simulink model "EfficiencySensitivityAnalysis"  (R2024b)
settings: Solver=FixedStepAuto  StartTime=0.0  StopTime=451.4  FixedStep=0.1  RelTol=1e-3
values from neighbouring files (symbols this model uses):
  GR = 6    [EfficiencySensitivityAnalysisParameters.m]
  mu_gb = 0.95    [EfficiencySensitivityAnalysisParameters.m]
  phi = 0    [EfficiencySensitivityAnalysisParameters.m]
  Tinit = 40    [EfficiencySensitivityAnalysisParameters.m]
  Tr = 0.33    [EfficiencySensitivityAnalysisParameters.m]
(part 3 of 3)

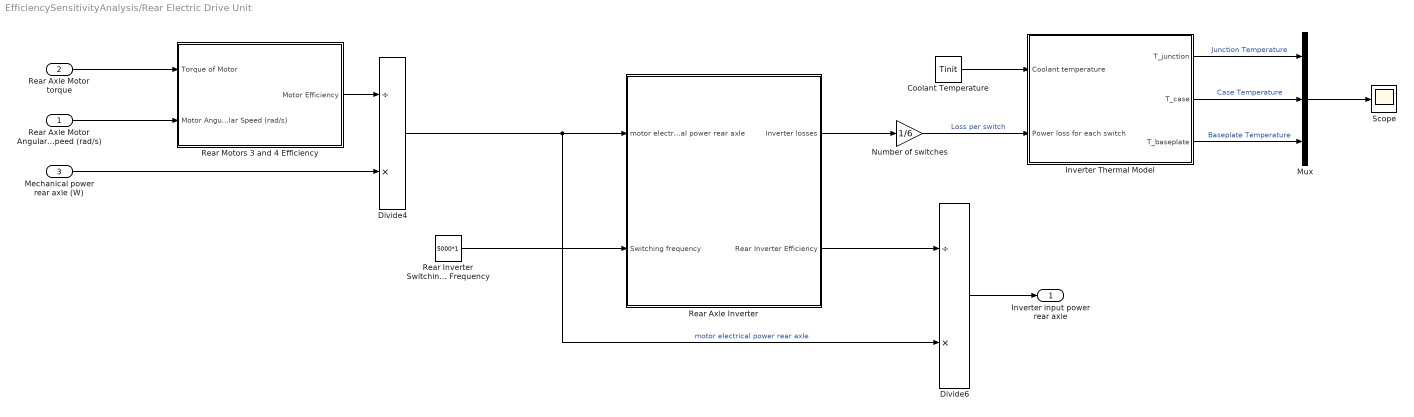
== system EfficiencySensitivityAnalysis/Rear Electric Drive Unit ==
  Rear Axle Motor Angular Speed (rad/s) : Inport
  Rear Axle Motor torque : Inport  Port=2
  Mechanical power rear axle (W) : Inport  Port=3
  Coolant Temperature : Constant  Value=Tinit
  Divide4 : Product  Inputs=/*
  Divide6 : Product  Inputs=/*
  Inverter Thermal Model : Subsystem
  Mux : Mux  Inputs=3
  Number of switches : Gain  Gain=1/6
  Rear Axle Inverter : Subsystem
  Rear Inverter Switching Frequency : Constant  Value=5000*1
  Rear Motors 3 and 4 Efficiency : Subsystem
  Scope : Scope
  Inverter input power rear axle : Outport
  wires:
  Rear Inverter Switching Frequency/1 -> Rear Axle Inverter/2(Switching frequency)
  Rear Axle Motor Angular Speed (rad/s)/1 -> Rear Motors 3 and 4 Efficiency/2(Motor Angular Speed (rad/s))
  Mechanical power rear axle (W)/1 -> Divide4/2
  Divide6/1 -> Inverter input power rear axle/1
  Rear Motors 3 and 4 Efficiency/1(Motor Efficiency) -> Divide4/1
  Rear Axle Motor torque/1 -> Rear Motors 3 and 4 Efficiency/1(Torque of Motor)
  Rear Axle Inverter/2(Rear Inverter Efficiency) -> Divide6/1
  Coolant Temperature/1 -> Inverter Thermal Model/1(Coolant temperature)
  Rear Axle Inverter/1(Inverter losses) -> Number of switches/1
  Number of switches/1 -> Inverter Thermal Model/2(Power loss for each switch)  "Loss per switch"
  Inverter Thermal Model/1(T_junction) -> Mux/1  "Junction Temperature"
  Inverter Thermal Model/2(T_case) -> Mux/2  "Case Temperature"
  Inverter Thermal Model/3(T_baseplate) -> Mux/3  "Baseplate Temperature"
  Mux/1 -> Scope/1
  Divide4/1 -> Divide6/2, Rear Axle Inverter/1(motor electrical power rear axle)  "motor electrical power rear axle"

== system EfficiencySensitivityAnalysis/Battery/Battery Thermal Model ==
  In1 : Inport
  In2 : Inport  Port=2
  1/R_thjc : Gain  Gain=1/0.15
  C_th_junction : Gain  Gain=1/(25*10^4)
  Integrator : Integrator  InitialCondition=25
  Subtract : Sum  Inputs=+-
  Subtract1 : Sum  Inputs=-+
  Battery  temperature : Outport
  wires:
  In2/1 -> Subtract1/2
  C_th_junction/1 -> Integrator/1
  Subtract1/1 -> C_th_junction/1
  Integrator/1 -> Battery  temperature/1, Subtract/1  "Battery  temperature"
  In1/1 -> Subtract/2
  Subtract/1 -> 1/R_thjc/1
  1/R_thjc/1 -> Subtract1/1

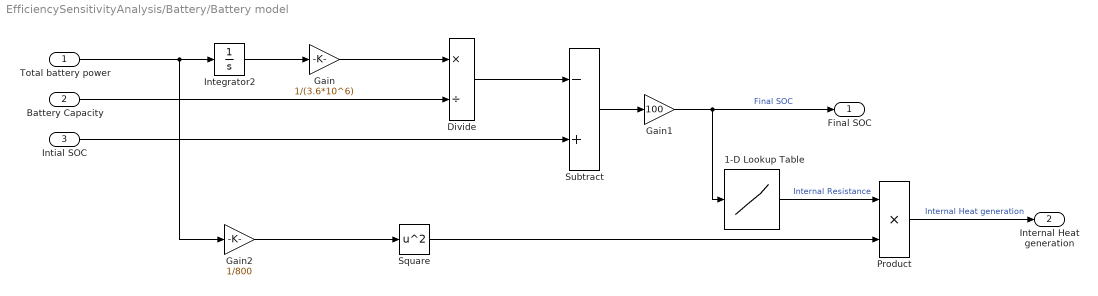
== system EfficiencySensitivityAnalysis/Battery/Battery model ==
  Total battery power : Inport
  Battery Capacity : Inport  Port=2
  Intial SOC : Inport  Port=3
  1-D Lookup Table : Lookup_n-D  NumberOfTableDimensions=1  BreakpointsForDimension1=[1 10 20 30 40 50 60 70 80 90 99]  Table=[0.038 0.037 0.0365 0.036 0.0357 0.035 0.0347 0.0343 0.0342 0.0342 0.035]  InternalRulePriority=Speed  RndMeth=Simplest
  Divide : Product  Inputs=*/
  Gain : Gain  Gain=1/(3.6*10^6)
  Gain1 : Gain  Gain=100
  Gain2 : Gain  Gain=1/800
  Integrator2 : Integrator
  Product : Product
  Square : Math  Operator=square
  Subtract : Sum  Inputs=-+
  Final SOC : Outport
  Internal Heat generation : Outport  Port=2
  wires:
  Total battery power/1 -> Gain2/1, Integrator2/1
  Gain1/1 -> 1-D Lookup Table/1, Final SOC/1  "Final SOC"
  Gain/1 -> Divide/1
  Subtract/1 -> Gain1/1
  Battery Capacity/1 -> Divide/2
  Integrator2/1 -> Gain/1
  1-D Lookup Table/1 -> Product/1  "Internal Resistance"
  Square/1 -> Product/2
  Product/1 -> Internal Heat generation/1  "Internal Heat generation"
  Gain2/1 -> Square/1
  Divide/1 -> Subtract/1
  Intial SOC/1 -> Subtract/2

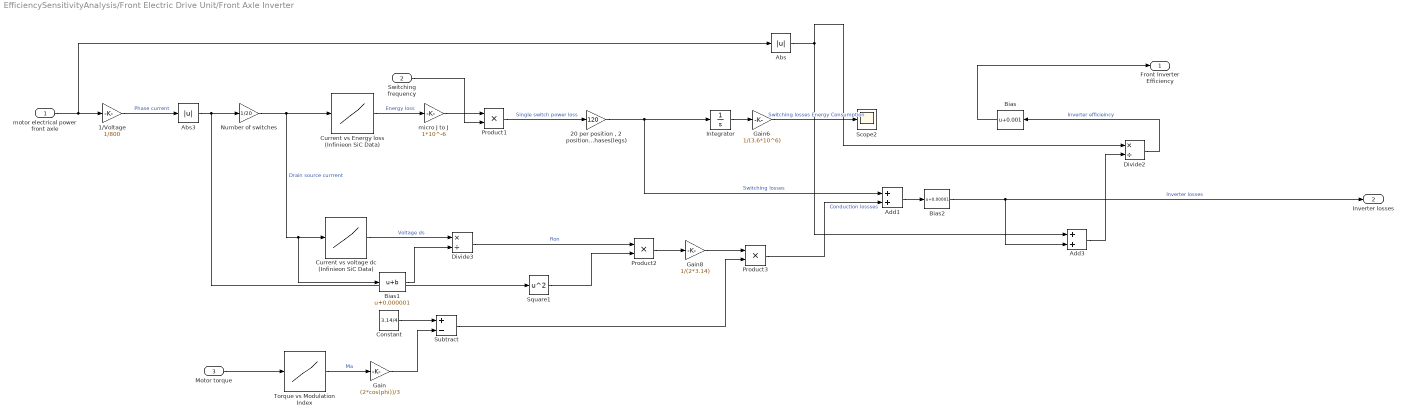
== system EfficiencySensitivityAnalysis/Front Electric Drive Unit/Front Axle Inverter ==
  motor electrical power front axle : Inport
  Switching frequency : Inport  Port=2
  Motor torque : Inport  Port=3
  1/Voltage : Gain  Gain=1/800
  "20 per position , 2 positions and 3 phases(legs)" : Gain  Gain=120
  Abs : Abs  SaturateOnIntegerOverflow=off
  Abs3 : Abs  SaturateOnIntegerOverflow=off
  Add1 : Sum
  Add3 : Sum
  Bias : Bias  Bias=0.001  SaturateOnIntegerOverflow=off
  Bias1 : Bias  Bias=0.000001  SaturateOnIntegerOverflow=off
  Bias2 : Bias  Bias=0.00001  SaturateOnIntegerOverflow=off
  Constant : Constant  Value=3.14/4
  Current vs Energy loss (Infinieon SiC Data) : Lookup_n-D  NumberOfTableDimensions=1  BreakpointsForDimension1=[0;5;10;15;20;25;30;35;40;45;50]  Table=[0;250;300;380;500;600;750;900;1050;1200;1400]  InternalRulePriority=Speed  RndMeth=Simplest
  Current vs voltage dc (Infinieon SiC Data) : Lookup_n-D  NumberOfTableDimensions=1  BreakpointsForDimension1=[20;40;60;80;110]  Table=[1;2;5;8;20]  InternalRulePriority=Speed  RndMeth=Simplest
  Divide2 : Product  Inputs=*/
  Divide3 : Product  Inputs=*/
  Gain : Gain  Gain=(2*cos(phi))/3
  Gain6 : Gain  Gain=1/(3.6*10^6)
  Gain8 : Gain  Gain=1/(2*3.14)
  Integrator : Integrator
  Number of switches : Gain  Gain=1/20
  Product1 : Product
  Product2 : Product
  Product3 : Product
  Scope2 : Scope
  Square1 : Math  Operator=square
  Subtract : Sum  Inputs=+-
  Torque vs Modulation Index : Lookup_n-D  NumberOfTableDimensions=1  BreakpointsForDimension1=[0;100;200;300;400]  Table=[0.3;0.5;0.7;0.8;0.95]  InternalRulePriority=Speed  RndMeth=Simplest
  micro J to J : Gain  Gain=1*10^-6
  Front Inverter Efficiency : Outport
  Inverter losses : Outport  Port=2
  wires:
  Bias/1 -> Front Inverter Efficiency/1
  Switching frequency/1 -> Product1/2
  Integrator/1 -> Gain6/1
  Current vs Energy loss (Infinieon SiC Data)/1 -> micro J to J/1  "Energy loss"
  motor electrical power front axle/1 -> Abs/1, 1/Voltage/1
  Abs/1 -> Divide2/1, Add3/1
  Gain/1 -> Subtract/2
  Add1/1 -> Bias2/1
  Constant/1 -> Subtract/1
  Square1/1 -> Product2/2
  Torque vs Modulation Index/1 -> Gain/1  "Ma"
  Motor torque/1 -> Torque vs Modulation Index/1
  Divide3/1 -> Product2/1  "Ron"
  Divide2/1 -> Bias/1  "Inverter efficieincy"
  Current vs voltage dc (Infinieon SiC Data)/1 -> Divide3/1  "Voltage ds"
  Subtract/1 -> Product3/2
  Number of switches/1 -> Bias1/1, Current vs voltage dc (Infinieon SiC Data)/1, Current vs Energy loss (Infinieon SiC Data)/1  "Drain source currrent"
  Product3/1 -> Add1/2  "Conduction lossses"
  Product2/1 -> Gain8/1
  Add3/1 -> Divide2/2
  Product1/1 -> "20 per position , 2 positions and 3 phases(legs)"/1  "Single switch power loss"
  "20 per position , 2 positions and 3 phases(legs)"/1 -> Integrator/1, Add1/1  "Switching losses"
  micro J to J/1 -> Product1/1
  1/Voltage/1 -> Abs3/1  "Phase current"
  Gain8/1 -> Product3/1
  Bias1/1 -> Divide3/2
  Gain6/1 -> Scope2/1  "Switching losses Energy Consumption"
  Bias2/1 -> Inverter losses/1, Add3/2  "Inverter losses"
  Abs3/1 -> Square1/1, Number of switches/1

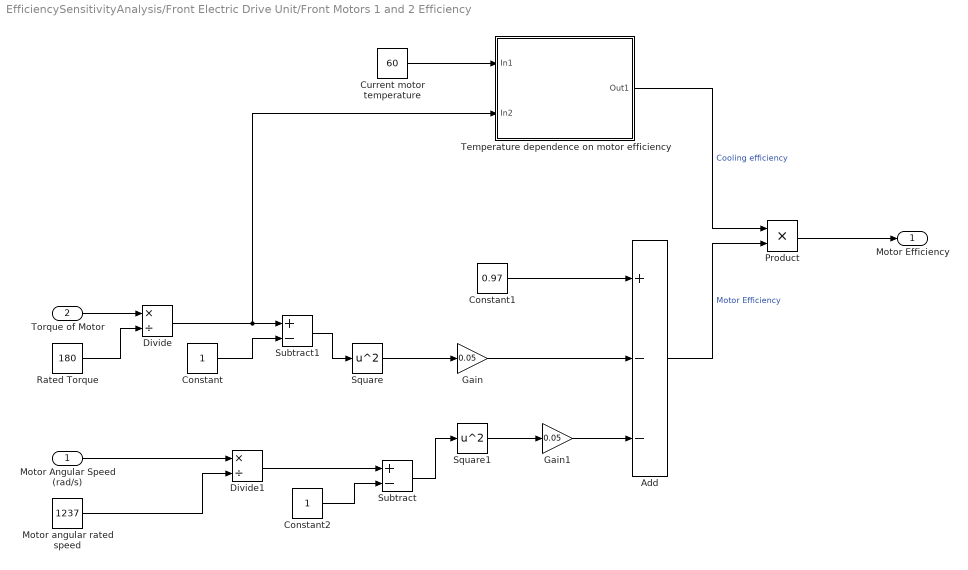
== system EfficiencySensitivityAnalysis/Front Electric Drive Unit/Front Motors 1 and 2 Efficiency  ==
  Motor Angular Speed (rad/s) : Inport
  Torque of Motor : Inport  Port=2
  Add : Sum  Inputs=+--
  Constant : Constant
  Constant1 : Constant  Value=0.97
  Constant2 : Constant
  Current motor temperature : Constant  Value=60
  Divide : Product  Inputs=*/
  Divide1 : Product  Inputs=*/
  Gain : Gain  Gain=0.05
  Gain1 : Gain  Gain=0.05
  Motor angular rated speed : Constant  Value=1237
  Product : Product
  Rated Torque : Constant  Value=180
  Square : Math  Operator=square
  Square1 : Math  Operator=square
  Subtract : Sum  Inputs=+-
  Subtract1 : Sum  Inputs=+-
  Temperature dependence on motor efficiency : Subsystem
  Motor Efficiency : Outport
  wires:
  Constant1/1 -> Add/1
  Square1/1 -> Gain1/1
  Gain/1 -> Add/2
  Constant2/1 -> Subtract/2
  Gain1/1 -> Add/3
  Subtract/1 -> Square1/1
  Motor angular rated speed/1 -> Divide1/2
  Torque of Motor/1 -> Divide/1
  Divide/1 -> Temperature dependence on motor efficiency/2(In2), Subtract1/1
  Square/1 -> Gain/1
  Rated Torque/1 -> Divide/2
  Subtract1/1 -> Square/1
  Current motor temperature/1 -> Temperature dependence on motor efficiency/1(In1)
  Divide1/1 -> Subtract/1
  Constant/1 -> Subtract1/2
  Add/1 -> Product/2  "Motor Efficiency"
  Temperature dependence on motor efficiency/1(Out1) -> Product/1  "Cooling efficiency"
  Motor Angular Speed (rad/s)/1 -> Divide1/1
  Product/1 -> Motor Efficiency/1

== system EfficiencySensitivityAnalysis/Front Electric Drive Unit/Inverter Thermal Model ==
  Coolant temperature : Inport
  Power loss for each switch : Inport  Port=2
  Base plate thermal model : Subsystem
  Case thermal model : Subsystem
  Junction thermal model : Subsystem
  T_junction : Outport
  T_case : Outport  Port=2
  T_baseplate : Outport  Port=3
  wires:
  Junction thermal model/1(Junction temperature) -> Case thermal model/1(Junction temperature), T_junction/1
  Case thermal model/1(Case temperature) -> T_case/1, Base plate thermal model/1(Case temperature), Junction thermal model/1(Case temperature)
  Base plate thermal model/1(Baseplate temperature) -> T_baseplate/1, Case thermal model/2(Base plate temperature)
  Coolant temperature/1 -> Base plate thermal model/2(Coolant temperature)
  Power loss for each switch/1 -> Junction thermal model/2(Power loss for each switch)

== system EfficiencySensitivityAnalysis/Rear Electric Drive Unit/Inverter Thermal Model ==
  Coolant temperature : Inport
  Power loss for each switch : Inport  Port=2
  Base plate thermal model : Subsystem
  Case thermal model : Subsystem
  Junction thermal model : Subsystem
  T_junction : Outport
  T_case : Outport  Port=2
  T_baseplate : Outport  Port=3
  wires:
  Junction thermal model/1(Junction temperature) -> Case thermal model/1(Junction temperature), T_junction/1
  Case thermal model/1(Case temperature) -> T_case/1, Base plate thermal model/1(Case temperature), Junction thermal model/1(Case temperature)
  Base plate thermal model/1(Baseplate temperature) -> T_baseplate/1, Case thermal model/2(Base plate temperature)
  Coolant temperature/1 -> Base plate thermal model/2(Coolant temperature)
  Power loss for each switch/1 -> Junction thermal model/2(Power loss for each switch)

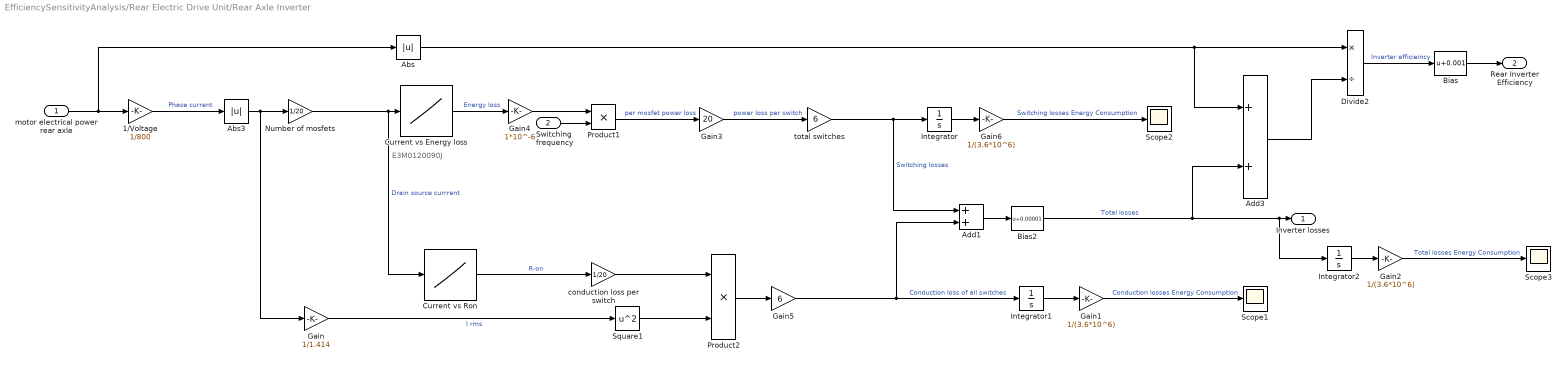
== system EfficiencySensitivityAnalysis/Rear Electric Drive Unit/Rear Axle Inverter ==
  note: E3M0120090J
  motor electrical power rear axle : Inport
  Switching frequency : Inport  Port=2
  1/Voltage : Gain  Gain=1/800
  Abs : Abs  SaturateOnIntegerOverflow=off
  Abs3 : Abs  SaturateOnIntegerOverflow=off
  Add1 : Sum
  Add3 : Sum
  Bias : Bias  Bias=0.001  SaturateOnIntegerOverflow=off
  Bias2 : Bias  Bias=0.00001  SaturateOnIntegerOverflow=off
  "Current vs Energy loss " : Lookup_n-D  NumberOfTableDimensions=1  BreakpointsForDimension1=[5;10;15;20;25;30]  Table=[21;26;32;40;55;70]  InternalRulePriority=Speed  RndMeth=Simplest
  "Current vs Ron " : Lookup_n-D  NumberOfTableDimensions=1  BreakpointsForDimension1=[5;10;15;20;25;30]  Table=[0.15;0.152;0.158;0.165;0.17;0.175]  InternalRulePriority=Speed  RndMeth=Simplest
  Divide2 : Product  Inputs=*/
  Gain : Gain  Gain=1/1.414
  Gain1 : Gain  Gain=1/(3.6*10^6)
  Gain2 : Gain  Gain=1/(3.6*10^6)
  Gain3 : Gain  Gain=20
  Gain4 : Gain  Gain=1*10^-6
  Gain5 : Gain  Gain=6
  Gain6 : Gain  Gain=1/(3.6*10^6)
  Integrator : Integrator
  Integrator1 : Integrator
  Integrator2 : Integrator
  Number of mosfets : Gain  Gain=1/20
  Product1 : Product
  Product2 : Product
  Scope1 : Scope
  Scope2 : Scope
  Scope3 : Scope
  Square1 : Math  Operator=square
  conduction loss per switch : Gain  Gain=1/20
  total switches : Gain  Gain=6
  Inverter losses : Outport
  Rear Inverter Efficiency : Outport  Port=2
  wires:
  Bias/1 -> Rear Inverter Efficiency/1
  Switching frequency/1 -> Product1/2
  Integrator/1 -> Gain6/1
  motor electrical power rear axle/1 -> Abs/1, 1/Voltage/1
  Abs/1 -> Divide2/1, Add3/1
  Add1/1 -> Bias2/1
  Square1/1 -> Product2/2
  Divide2/1 -> Bias/1  "Inverter efficieincy"
  Add3/1 -> Divide2/2
  Product1/1 -> Gain3/1  "per mosfet power loss"
  total switches/1 -> Integrator/1, Add1/1  "Switching losses"
  1/Voltage/1 -> Abs3/1  "Phase current"
  Gain6/1 -> Scope2/1  "Switching losses Energy Consumption"
  Abs3/1 -> Number of mosfets/1, Gain/1
  Integrator1/1 -> Gain1/1
  Gain1/1 -> Scope1/1  "Conduction losses Energy Consumption"
  Product2/1 -> Gain5/1
  Gain2/1 -> Scope3/1  "Total losses Energy Consumption"
  Integrator2/1 -> Gain2/1
  Bias2/1 -> Inverter losses/1, Integrator2/1, Add3/2  "Total losses"
  Gain/1 -> Square1/1  "I rms"
  Gain4/1 -> Product1/1
  Number of mosfets/1 -> "Current vs Ron "/1, "Current vs Energy loss "/1  "Drain source currrent"
  "Current vs Energy loss "/1 -> Gain4/1  "Energy loss"
  "Current vs Ron "/1 -> conduction loss per switch/1  "R-on"
  conduction loss per switch/1 -> Product2/1
  Gain5/1 -> Integrator1/1, Add1/2  "Conduction loss of all switches"
  Gain3/1 -> total switches/1  "power loss per switch"

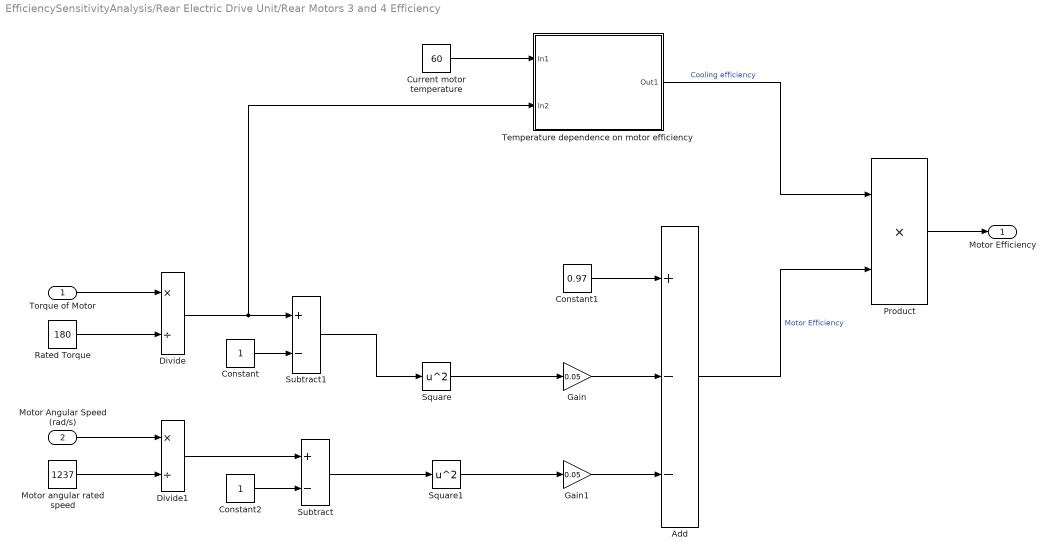
== system EfficiencySensitivityAnalysis/Rear Electric Drive Unit/Rear Motors 3 and 4 Efficiency ==
  Torque of Motor : Inport
  Motor Angular Speed (rad/s) : Inport  Port=2
  Add : Sum  Inputs=+--
  Constant : Constant
  Constant1 : Constant  Value=0.97
  Constant2 : Constant
  Current motor temperature : Constant  Value=60
  Divide : Product  Inputs=*/
  Divide1 : Product  Inputs=*/
  Gain : Gain  Gain=0.05
  Gain1 : Gain  Gain=0.05
  Motor angular rated speed : Constant  Value=1237
  Product : Product
  Rated Torque : Constant  Value=180
  Square : Math  Operator=square
  Square1 : Math  Operator=square
  Subtract : Sum  Inputs=+-
  Subtract1 : Sum  Inputs=+-
  Temperature dependence on motor efficiency : Subsystem
  Motor Efficiency : Outport
  wires:
  Torque of Motor/1 -> Divide/1
  Motor Angular Speed (rad/s)/1 -> Divide1/1
  Subtract/1 -> Square1/1
  Gain/1 -> Add/2
  Constant2/1 -> Subtract/2
  Divide1/1 -> Subtract/1
  Rated Torque/1 -> Divide/2
  Constant/1 -> Subtract1/2
  Constant1/1 -> Add/1
  Gain1/1 -> Add/3
  Motor angular rated speed/1 -> Divide1/2
  Square1/1 -> Gain1/1
  Square/1 -> Gain/1
  Subtract1/1 -> Square/1
  Divide/1 -> Temperature dependence on motor efficiency/2(In2), Subtract1/1
  Temperature dependence on motor efficiency/1(Out1) -> Product/1  "Cooling efficiency"
  Current motor temperature/1 -> Temperature dependence on motor efficiency/1(In1)
  Add/1 -> Product/2  "Motor Efficiency"
  Product/1 -> Motor Efficiency/1

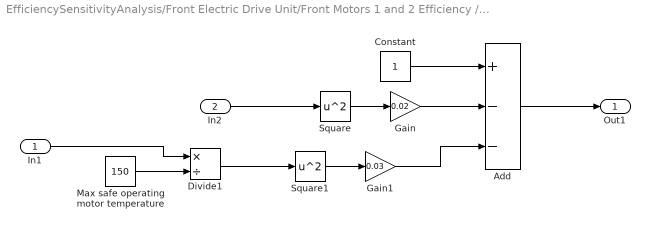
== system EfficiencySensitivityAnalysis/Front Electric Drive Unit/Front Motors 1 and 2 Efficiency /Temperature dependence on motor efficiency ==
  In1 : Inport
  In2 : Inport  Port=2
  Add : Sum  Inputs=+--
  Constant : Constant
  Divide1 : Product  Inputs=*/
  Gain : Gain  Gain=0.02
  Gain1 : Gain  Gain=0.03
  Max safe operating motor temperature : Constant  Value=150
  Square : Math  Operator=square
  Square1 : Math  Operator=square
  Out1 : Outport
  wires:
  Square/1 -> Gain/1
  Square1/1 -> Gain1/1
  In1/1 -> Divide1/1
  Divide1/1 -> Square1/1
  Add/1 -> Out1/1
  Gain1/1 -> Add/3
  Max safe operating motor temperature/1 -> Divide1/2
  Gain/1 -> Add/2
  Constant/1 -> Add/1
  In2/1 -> Square/1

== system EfficiencySensitivityAnalysis/Front Electric Drive Unit/Inverter Thermal Model/Base plate thermal model ==
  Case temperature : Inport
  Coolant temperature : Inport  Port=2
  1/R_thbs : Gain  Gain=1/0.03
  1/R_thcb : Gain  Gain=1/0.015
  Add : Sum  Inputs=+-
  Gain : Gain  Gain=1/100
  Integrator : Integrator  InitialCondition=Tinit
  Subtract : Sum  Inputs=+-
  Subtract1 : Sum  Inputs=+-
  Baseplate temperature : Outport
  wires:
  Integrator/1 -> Subtract/2, Baseplate temperature/1, Subtract1/1  "Baseplate temperature"
  1/R_thcb/1 -> Add/1
  Gain/1 -> Integrator/1
  Subtract/1 -> 1/R_thcb/1
  Case temperature/1 -> Subtract/1
  Coolant temperature/1 -> Subtract1/2
  Subtract1/1 -> 1/R_thbs/1
  1/R_thbs/1 -> Add/2
  Add/1 -> Gain/1

== system EfficiencySensitivityAnalysis/Front Electric Drive Unit/Inverter Thermal Model/Case thermal model ==
  Junction temperature : Inport
  Base plate temperature : Inport  Port=2
  1/R_thcb : Gain  Gain=1/0.015
  1/R_thjc : Gain  Gain=1/0.51
  Gain : Gain  Gain=1/20
  Integrator : Integrator  InitialCondition=Tinit
  Subtract : Sum  Inputs=+-
  Subtract1 : Sum  Inputs=+-
  Subtract2 : Sum  Inputs=+-
  Case temperature : Outport
  wires:
  Subtract1/1 -> Gain/1
  Integrator/1 -> Case temperature/1, Subtract2/1, Subtract/2  "Case temperature"
  Gain/1 -> Integrator/1
  Subtract/1 -> 1/R_thjc/1
  Base plate temperature/1 -> Subtract2/2
  Subtract2/1 -> 1/R_thcb/1
  1/R_thcb/1 -> Subtract1/2
  Junction temperature/1 -> Subtract/1
  1/R_thjc/1 -> Subtract1/1

== system EfficiencySensitivityAnalysis/Front Electric Drive Unit/Inverter Thermal Model/Junction thermal model ==
  Case temperature : Inport
  Power loss for each switch : Inport  Port=2
  1/R_thjc : Gain  Gain=1/0.25
  C_th_junction : Gain  Gain=1/6
  Integrator : Integrator  InitialCondition=Tinit
  Subtract : Sum  Inputs=+-
  Subtract1 : Sum  Inputs=-+
  Junction temperature : Outport
  wires:
  Integrator/1 -> Subtract/1, Junction temperature/1  "Junction temperature"
  C_th_junction/1 -> Integrator/1
  Subtract/1 -> 1/R_thjc/1
  Case temperature/1 -> Subtract/2
  1/R_thjc/1 -> Subtract1/1
  Power loss for each switch/1 -> Subtract1/2
  Subtract1/1 -> C_th_junction/1

== system EfficiencySensitivityAnalysis/Rear Electric Drive Unit/Inverter Thermal Model/Base plate thermal model ==
  Case temperature : Inport
  Coolant temperature : Inport  Port=2
  1/R_thbs : Gain  Gain=1/0.03
  1/R_thcb : Gain  Gain=1/0.015
  Add : Sum  Inputs=+-
  Gain : Gain  Gain=1/100
  Integrator : Integrator  InitialCondition=Tinit
  Subtract : Sum  Inputs=+-
  Subtract1 : Sum  Inputs=+-
  Baseplate temperature : Outport
  wires:
  Integrator/1 -> Subtract/2, Baseplate temperature/1, Subtract1/1  "Baseplate temperature"
  1/R_thcb/1 -> Add/1
  Gain/1 -> Integrator/1
  Subtract/1 -> 1/R_thcb/1
  Case temperature/1 -> Subtract/1
  Coolant temperature/1 -> Subtract1/2
  Subtract1/1 -> 1/R_thbs/1
  1/R_thbs/1 -> Add/2
  Add/1 -> Gain/1

== system EfficiencySensitivityAnalysis/Rear Electric Drive Unit/Inverter Thermal Model/Case thermal model ==
  Junction temperature : Inport
  Base plate temperature : Inport  Port=2
  1/R_thcb : Gain  Gain=1/0.015
  1/R_thjc : Gain  Gain=1/0.51
  Gain : Gain  Gain=1/20
  Integrator : Integrator  InitialCondition=Tinit
  Subtract : Sum  Inputs=+-
  Subtract1 : Sum  Inputs=+-
  Subtract2 : Sum  Inputs=+-
  Case temperature : Outport
  wires:
  Subtract1/1 -> Gain/1
  Integrator/1 -> Case temperature/1, Subtract2/1, Subtract/2  "Case temperature"
  Gain/1 -> Integrator/1
  Subtract/1 -> 1/R_thjc/1
  Base plate temperature/1 -> Subtract2/2
  Subtract2/1 -> 1/R_thcb/1
  1/R_thcb/1 -> Subtract1/2
  Junction temperature/1 -> Subtract/1
  1/R_thjc/1 -> Subtract1/1

== system EfficiencySensitivityAnalysis/Rear Electric Drive Unit/Inverter Thermal Model/Junction thermal model ==
  Case temperature : Inport
  Power loss for each switch : Inport  Port=2
  1/R_thjc : Gain  Gain=1/0.15
  C_th_junction : Gain  Gain=1/10
  Integrator : Integrator  InitialCondition=Tinit
  Subtract : Sum  Inputs=+-
  Subtract1 : Sum  Inputs=-+
  Junction temperature : Outport
  wires:
  Integrator/1 -> Subtract/1, Junction temperature/1  "Junction temperature"
  C_th_junction/1 -> Integrator/1
  Subtract/1 -> 1/R_thjc/1
  Case temperature/1 -> Subtract/2
  1/R_thjc/1 -> Subtract1/1
  Power loss for each switch/1 -> Subtract1/2
  Subtract1/1 -> C_th_junction/1

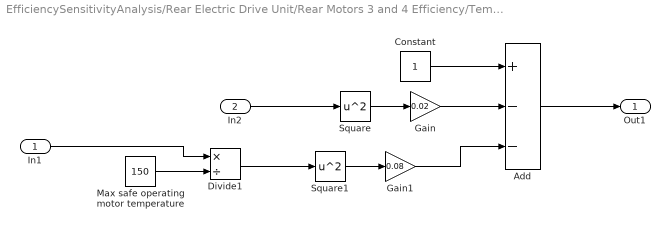
== system EfficiencySensitivityAnalysis/Rear Electric Drive Unit/Rear Motors 3 and 4 Efficiency/Temperature dependence on motor efficiency ==
  In1 : Inport
  In2 : Inport  Port=2
  Add : Sum  Inputs=+--
  Constant : Constant
  Divide1 : Product  Inputs=*/
  Gain : Gain  Gain=0.02
  Gain1 : Gain  Gain=0.08
  Max safe operating motor temperature : Constant  Value=150
  Square : Math  Operator=square
  Square1 : Math  Operator=square
  Out1 : Outport
  wires:
  Square/1 -> Gain/1
  Square1/1 -> Gain1/1
  In1/1 -> Divide1/1
  Divide1/1 -> Square1/1
  Add/1 -> Out1/1
  Gain1/1 -> Add/3
  Max safe operating motor temperature/1 -> Divide1/2
  Gain/1 -> Add/2
  Constant/1 -> Add/1
  In2/1 -> Square/1
